simulink model "AC1P1_model"  (R2025b)
settings: Solver=VariableStepAuto  StartTime=0.0  StopTime=10.0  MaxStep=0.05  RelTol=1e-3
values from neighbouring files (symbols this model uses):
  c = 5    [AC1P1_script.m]
  k = 125    [AC1P1_script.m]
  m = 5    [AC1P1_script.m]
libraries: simulink x1
settings Model: Creator=micha  LastModifiedBy=micha

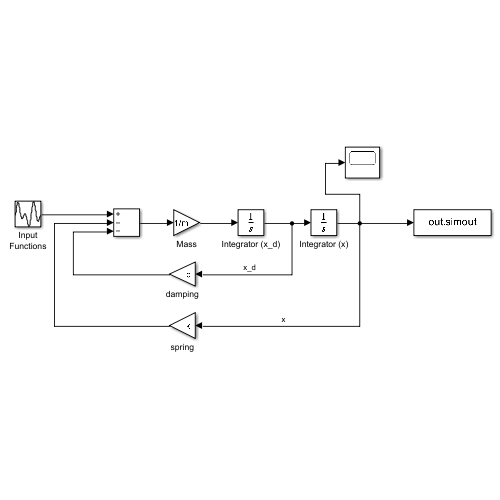
[thumbnail: Simulink's stored preview of the top-level diagram]
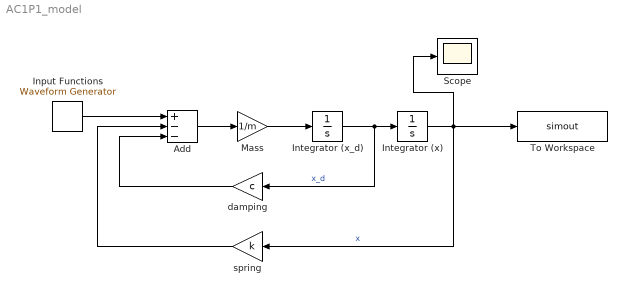
== system AC1P1_model ==
  Add : Sum  Inputs=+--
  Input Functions : simulink/Sources/Waveform Generator  OutMin=[]  OutMax=[]  OutDataTypeStr=double  SelectedSignal=1  Signals=step(1,0,1)#sin(1,w,0)  BlockNames=MultiportSwitch_bb3abd99e6f7470#MultiportSwitch_ad21b82065af415  SampleTime=0.1
  Integrator (x) : Integrator
  Integrator (x_d) : Integrator
  Mass : Gain  Gain=1/m
  Scope : Scope
      settings: ActiveDisplayYMinimum=-0.0047806078447998508  ActiveDisplayYMaximum=0.0088124947302039309
  To Workspace : ToWorkspace  VariableName=simout  SaveFormat=Timeseries  SampleTime=-1
  damping : Gain  Gain=c
  spring : Gain  Gain=k
  wires:
  Add/1 -> Mass/1
  damping/1 -> Add/3
  spring/1 -> Add/2
  Mass/1 -> Integrator (x_d)/1
  Integrator (x_d)/1 -> damping/1, Integrator (x)/1  "x_d"
  Integrator (x)/1 -> To Workspace/1, Scope/1, spring/1  "x"
  Input Functions/1 -> Add/1
